simulink model "model6"  (R2020b)
settings: Solver=VariableStepAuto  StartTime=0.0  StopTime=60.0  MaxStep=1e-2  RelTol=1e-3
undefined symbols (not defined in the file): model6a
libraries: simulink x1
settings Model: Creator=swarn  LastModifiedBy=swarn

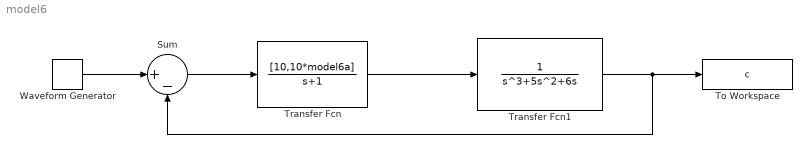
== system model6 ==
  Sum : Sum  Inputs=|+-
  To Workspace : ToWorkspace  VariableName=c  SaveFormat=Timeseries  SampleTime=-1
  Transfer Fcn : TransferFcn  Numerator=[10,10*model6a]  Denominator=[1 1]
  Transfer Fcn1 : TransferFcn  Denominator=[1,5,6,0]
  Waveform Generator : simulink/Sources/Waveform Generator  OutMin=[]  OutMax=[]  OutDataTypeStr=double  SelectedSignal=1  Signals=step(0,0,1)  BlockNames=MultiportSwitch_77ad4a2251064ef  SampleTime=0.1
  wires:
  Transfer Fcn/1 -> Transfer Fcn1/1
  Transfer Fcn1/1 -> To Workspace/1, Sum/2
  Sum/1 -> Transfer Fcn/1
  Waveform Generator/1 -> Sum/1
